simulink model "task5"  (R2022a)
settings: Solver=FixedStepAuto  StartTime=0.0  StopTime=1.5  FixedStep=0.001  RelTol=1e-3
values from neighbouring files (symbols this model uses):
  Anew = A*0.8    [Matlabfileassign2.m]
  B = [1 0 0 ... (first row only)    [Matlabfileassign2.m]
  C = [1 0 0 ... (first row only)    [Matlabfileassign2.m]
  K_i_tilde = inv(K_s)    [Matlabfileassign2.m]
  K_p_tilde = inv(K_s)    [Matlabfileassign2.m]
settings Model: Creator=Abdur Rafay  LastModifiedBy=Abdur Rafay

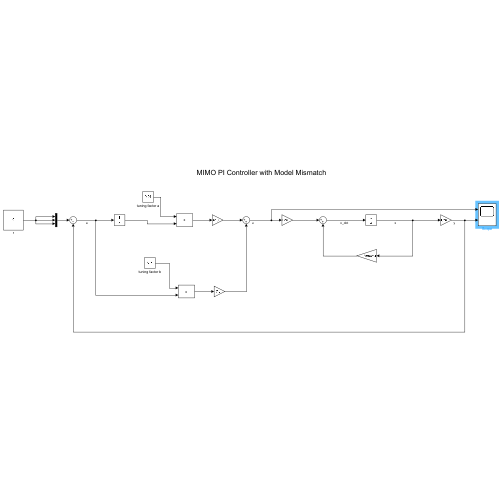
[thumbnail: Simulink's stored preview of the top-level diagram]
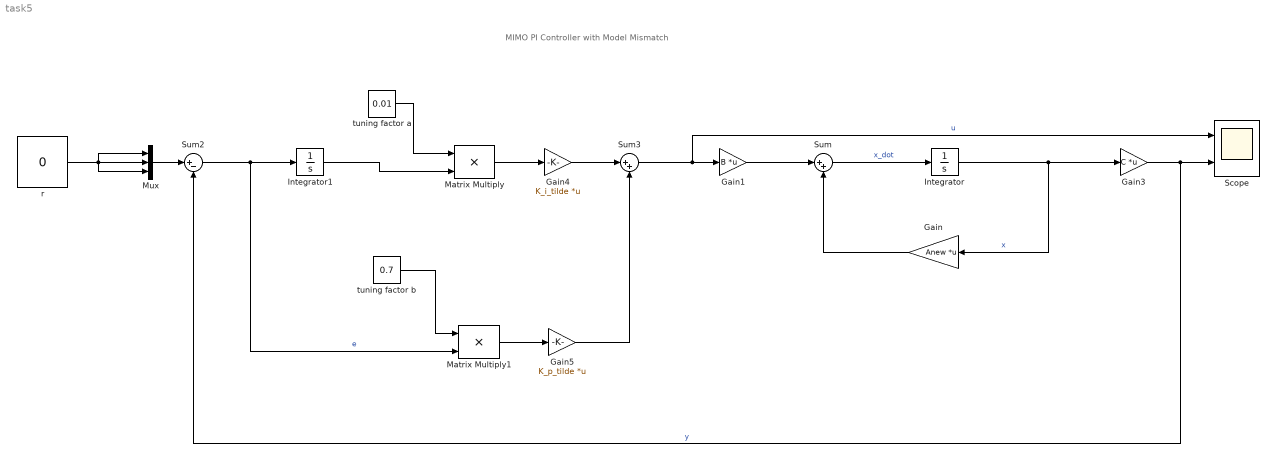
== system task5 ==
  note: MIMO PI Controller with Model Mismatch
  Gain : Gain  Gain=Anew  Multiplication=Matrix(K*u)
  Gain1 : Gain  Gain=B  Multiplication=Matrix(K*u)
  Gain3 : Gain  Gain=C  Multiplication=Matrix(K*u)
  Gain4 : Gain  Gain=K_i_tilde  Multiplication=Matrix(K*u)
  Gain5 : Gain  Gain=K_p_tilde  Multiplication=Matrix(K*u)
  Integrator : Integrator  InitialCondition=[1 1 1]
  Integrator1 : Integrator
  Matrix Multiply : Product
  Matrix Multiply1 : Product
  Mux : Mux  Inputs=3
  Scope : Scope  NumInputPorts=2
  Sum : Sum  Inputs=|++
  Sum2 : Sum  Inputs=|+-
  Sum3 : Sum  Inputs=|++
  r : Constant  Value=0
  tuning factor a : Constant  Value=0.01
  tuning factor b : Constant  Value=0.7
  wires:
  r/1 -> Mux/3, Mux/2, Mux/1
  Integrator1/1 -> Matrix Multiply/2
  Gain1/1 -> Sum/1
  Gain3/1 -> Scope/2, Sum2/2  "y"
  Integrator/1 -> Gain/1, Gain3/1  "x"
  Sum3/1 -> Scope/1, Gain1/1  "u"
  Sum/1 -> Integrator/1  "x_dot"
  tuning factor a/1 -> Matrix Multiply/1
  Gain/1 -> Sum/2
  Matrix Multiply1/1 -> Gain5/1
  Gain4/1 -> Sum3/1
  Matrix Multiply/1 -> Gain4/1
  tuning factor b/1 -> Matrix Multiply1/1
  Mux/1 -> Sum2/1
  Gain5/1 -> Sum3/2
  Sum2/1 -> Matrix Multiply1/2, Integrator1/1  "e"
